simulink model "esercitazione_8_sistema_sim"  (Simulink 8.5)
settings: Solver=ode45  StartTime=0.0  StopTime=30  RelTol=1e-3
values from neighbouring files (symbols this model uses):
  G = (K/(tau*s + 1))*exp(-L*s)    [lez8.m]
  PI1d = c2d(PI1, Ts, 'tustin')    [lez8.m]
  PID2d = c2d(PID2, Ts, 'tustin')    [lez8.m]
  Ts = 1/100    (= 0.01)    [lez8.m]
settings Model: Creator=claudio  LastModifiedBy=lezione  CovSFcnEnable=off
settings DataIOCC: SignalLoggingSaveFormat=Dataset
settings OptimizationCC: ExpressionDepthLimit=128
settings DebuggingCC: UnderspecifiedInitializationDetection=Simplified  MergeDetectMultiDrivingBlocksExec=error  SolverPrmCheckMsg=warning  FcnCallInpInsideContextMsg=EnableAllAsError  StateNameClashWarn=none
settings GRTTargetCC: CombineOutputUpdateFcns=on  GRTInterface=off

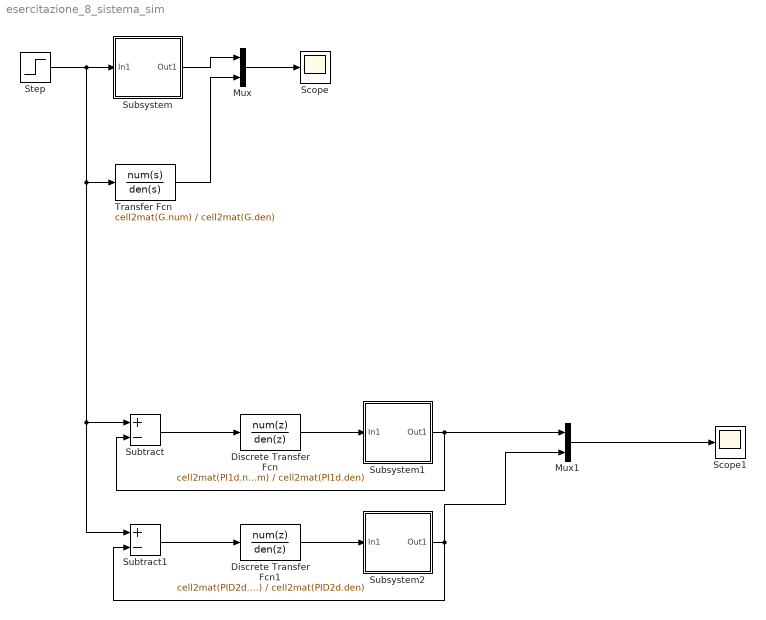
== system esercitazione_8_sistema_sim ==
  Discrete Transfer Fcn : DiscreteTransferFcn  Numerator=cell2mat(PI1d.num)  Denominator=cell2mat(PI1d.den)  SampleTime=Ts
  Discrete Transfer Fcn1 : DiscreteTransferFcn  Numerator=cell2mat(PID2d.num)  Denominator=cell2mat(PID2d.den)  SampleTime=Ts
  Mux : Mux  Inputs=2
  Mux1 : Mux  Inputs=2
  Scope : Scope
  Scope1 : Scope
      settings: MaxDataPoints=50000
  Step : Step  SampleTime=0
  Subsystem : Subsystem
  Subsystem1 : Subsystem
  Subsystem2 : Subsystem
  Subtract : Sum  Inputs=+-
  Subtract1 : Sum  Inputs=+-
  Transfer Fcn : TransferFcn  Numerator=cell2mat(G.num)  Denominator=cell2mat(G.den)
  wires:
  Step/1 -> Subtract1/1, Subtract/1, Transfer Fcn/1, Subsystem/1(In1)
  Transfer Fcn/1 -> Mux/2
  Subsystem/1(Out1) -> Mux/1
  Mux/1 -> Scope/1
  Discrete Transfer Fcn/1 -> Subsystem1/1(In1)
  Subtract/1 -> Discrete Transfer Fcn/1
  Subsystem1/1(Out1) -> Mux1/1, Subtract/2
  Subtract1/1 -> Discrete Transfer Fcn1/1
  Discrete Transfer Fcn1/1 -> Subsystem2/1(In1)
  Subsystem2/1(Out1) -> Mux1/2, Subtract1/2
  Mux1/1 -> Scope1/1

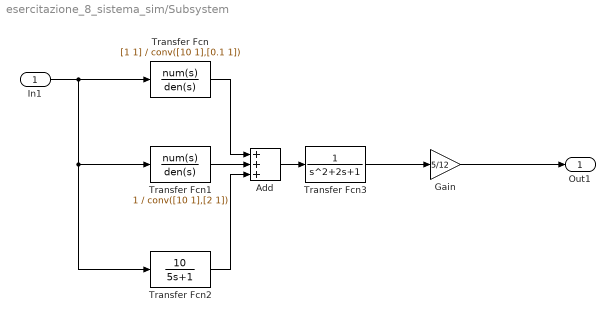
== system esercitazione_8_sistema_sim/Subsystem ==
  In1 : Inport
  Add : Sum  Inputs=+++
  Gain : Gain  Gain=5/12
  Transfer Fcn : TransferFcn  Numerator=[1 1]  Denominator=conv([10 1],[0.1 1])
  Transfer Fcn1 : TransferFcn  Numerator=1  Denominator=conv([10 1],[2 1])
  Transfer Fcn2 : TransferFcn  Numerator=10  Denominator=[5 1]
  Transfer Fcn3 : TransferFcn  Numerator=1
  Out1 : Outport
  wires:
  In1/1 -> Transfer Fcn2/1, Transfer Fcn1/1, Transfer Fcn/1
  Transfer Fcn1/1 -> Add/2
  Transfer Fcn/1 -> Add/1
  Add/1 -> Transfer Fcn3/1
  Transfer Fcn2/1 -> Add/3
  Transfer Fcn3/1 -> Gain/1
  Gain/1 -> Out1/1

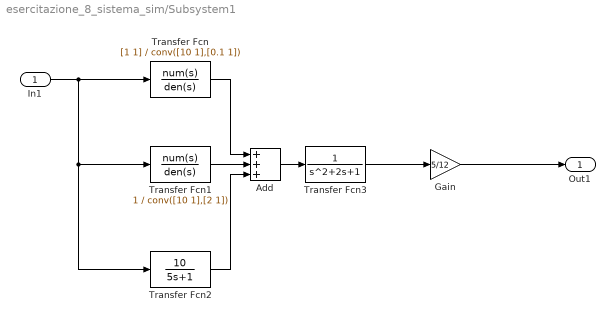
== system esercitazione_8_sistema_sim/Subsystem1 ==
  In1 : Inport
  Add : Sum  Inputs=+++
  Gain : Gain  Gain=5/12
  Transfer Fcn : TransferFcn  Numerator=[1 1]  Denominator=conv([10 1],[0.1 1])
  Transfer Fcn1 : TransferFcn  Numerator=1  Denominator=conv([10 1],[2 1])
  Transfer Fcn2 : TransferFcn  Numerator=10  Denominator=[5 1]
  Transfer Fcn3 : TransferFcn  Numerator=1
  Out1 : Outport
  wires:
  In1/1 -> Transfer Fcn2/1, Transfer Fcn1/1, Transfer Fcn/1
  Transfer Fcn1/1 -> Add/2
  Transfer Fcn/1 -> Add/1
  Add/1 -> Transfer Fcn3/1
  Transfer Fcn2/1 -> Add/3
  Transfer Fcn3/1 -> Gain/1
  Gain/1 -> Out1/1

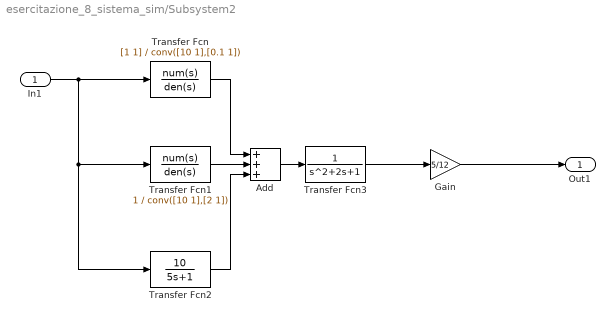
== system esercitazione_8_sistema_sim/Subsystem2 ==
  In1 : Inport
  Add : Sum  Inputs=+++
  Gain : Gain  Gain=5/12
  Transfer Fcn : TransferFcn  Numerator=[1 1]  Denominator=conv([10 1],[0.1 1])
  Transfer Fcn1 : TransferFcn  Numerator=1  Denominator=conv([10 1],[2 1])
  Transfer Fcn2 : TransferFcn  Numerator=10  Denominator=[5 1]
  Transfer Fcn3 : TransferFcn  Numerator=1
  Out1 : Outport
  wires:
  In1/1 -> Transfer Fcn2/1, Transfer Fcn1/1, Transfer Fcn/1
  Transfer Fcn1/1 -> Add/2
  Transfer Fcn/1 -> Add/1
  Add/1 -> Transfer Fcn3/1
  Transfer Fcn2/1 -> Add/3
  Transfer Fcn3/1 -> Gain/1
  Gain/1 -> Out1/1
